simulink model "mqam_2020a"  (R2020a)
settings: Solver=VariableStepAuto  StartTime=0.0  StopTime=10  RelTol=1e-3
PreLoadFcn:
  | %%% model parameters %%%
  | 
  | Rb = 10e6; % bit rate
  | Tb = 1/Rb; % bit interval
  | 
  | M = 256; % constelation alphabet
  | Nb = log2(M); % number of bit per symbol
  | 
  | Rsy = Rb/Nb; % symbol rate
  | Tsy = 1/Rsy; % symbol time
  | 
  | N = 100; % number of samples per symbol
  | 
  | Rsamp = N*Rsy; % sampling rate
  | Tsamp = 1/Rsamp; % samping interval
  | 
  | fc = 1/(4*Tsamp); % carrier frequency
  | 
  | Eg = 5; % baseband pulse shaping energy
  | 
  | %%% gray code mapper %%%
  | 
  | gray_codes = get_gray_codes(Nb/2);
  | 
  | gray_cont = containers.Map % container
  | for i=1:size(gray_codes,2)
  |   binary_str = num2str(flip(gray_codes(:,i)'));
  |   binary_str(binary_str == ' ') = '';
  |   gray_cont(binary_str) = (i-1)*2 - (sqrt(M) - 1);
  | end
  | 
  | %%% define the basbase shaping filter gain %%%
  | aux = rcosdesign(0.2, 4, N, 'normal');
  | Kg = 1/sqrt(trapz(Tsamp, aux.^2)); % filter gain so that the filter energy be normalized to unity
InitFcn:
  | phi = 0; % phase offset
undefined symbols (not defined in the file or in its folder): DiscIntNeverNeededParam, magnitude
libraries: dspsrcs4 x2, commchan3 x1, commfilt2 x1, commrandsrc3 x1, dsparch4 x1, commsink2 x1
settings Model: Creator=tapyu  LastModifiedBy=tapyu
settings DebuggingCC: UnconnectedInputMsg=none  UnconnectedOutputMsg=none  UnconnectedLineMsg=none  SFMachineParentedDataDiag=error

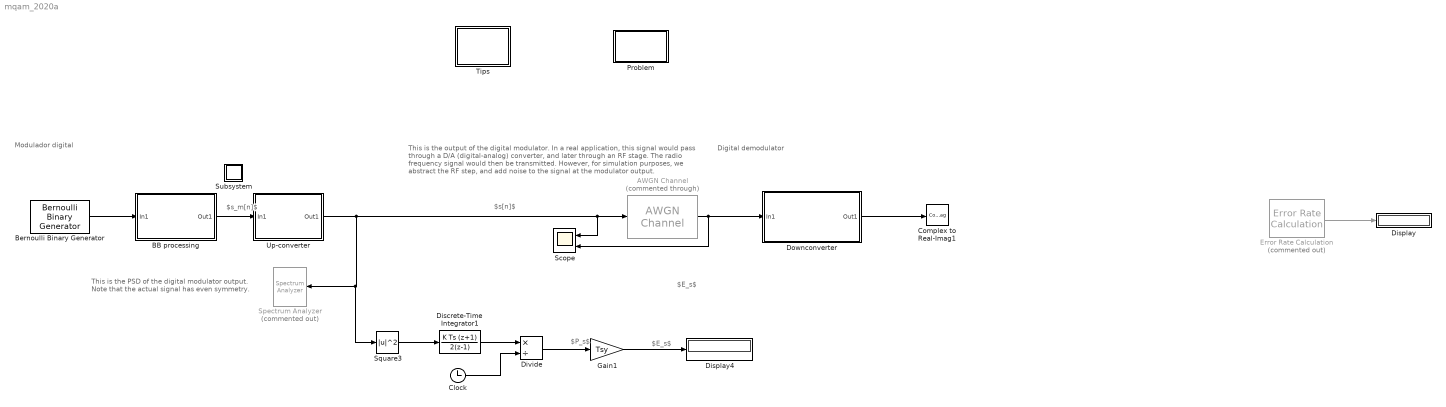
== system mqam_2020a ==
  note: Digital demodulator
  note: This is the output of the digital modulator. In a real application, this signal would
      | pass through a D/A (digital-analog) converter, and later through an RF stage.
      | The radio frequency signal would then be transmitted. However, for simulation
      | purposes, we abstract the RF step, and add noise to the signal at the modulator
      | output.
  note: $s[n]$
  note: This is the PSD of the digital modulator output.
      | Note that the actual signal has even symmetry.
  note: Modulador digital
  note: $s_m[n]$
  note: $E_s$
  note: $P_s$
  note: $E_s$
  AWGN Channel : commchan3/AWGN Channel  Commented=through  InputProcessing=Columns as channels (frame based)  seed=67  noiseMode="Signal to noise ratio  (Eb/No)"  EbNodB=10  EsNodB=10  SNRdB=10  bitsPerSym=sqrt(M)  Ps=1  Tsym=Tb  variance=1
  BB processing : Subsystem
  Bernoulli Binary Generator : commrandsrc3/Bernoulli Binary Generator  ProbabilityOfZero=0.5  SeedSource=Auto  Seed=0  SampleTime=Tb  SamplesPerFrame=1  OutputDataType=double  SimulateUsing=Interpreted execution
  Clock : Clock
  Complex to Real-Imag1 : ComplexToRealImag
  Discrete-Time Integrator1 : DiscreteIntegrator  IntegratorMethod=Integration: Trapezoidal  SampleTime=-1  ICPrevOutput=DiscIntNeverNeededParam  ICPrevScaledInput=DiscIntNeverNeededParam
  Display : Display
  Display4 : Display
  Divide : Product  Inputs=*/
  Downconverter : Subsystem
  Error Rate Calculation : commsink2/Error Rate Calculation  Commented=on  N=0  st_delay=0  cp_mode=Entire frame  subframe=[]  PMode=Port  WsName=ErrorVec  RsMode2=off  stop=off  numErr=100  maxBits=1e6
  Gain1 : Gain  Gain=Tsy
  Problem : Subsystem
  Scope : Scope  NumInputPorts=2
  Spectrum Analyzer : SpectrumAnalyzer  Commented=on
  Square3 : Math  Operator=magnitude^2  SaturateOnIntegerOverflow=on
  Subsystem : Subsystem
  Tips : Subsystem
  Up-converter : Subsystem
  wires:
  BB processing/1(Out1) -> Up-converter/1(In1)
  AWGN Channel/1 -> Downconverter/1(In1), Scope/2
  Error Rate Calculation/1 -> Display/1
  Downconverter/1(Out1) -> Complex to Real-Imag1/1
  Bernoulli Binary Generator/1 -> BB processing/1(In1)
  Gain1/1 -> Display4/1
  Clock/1 -> Divide/2
  Divide/1 -> Gain1/1
  Discrete-Time Integrator1/1 -> Divide/1
  Up-converter/1(Out1) -> Square3/1, Spectrum Analyzer/1, Scope/1, AWGN Channel/1
  Square3/1 -> Discrete-Time Integrator1/1

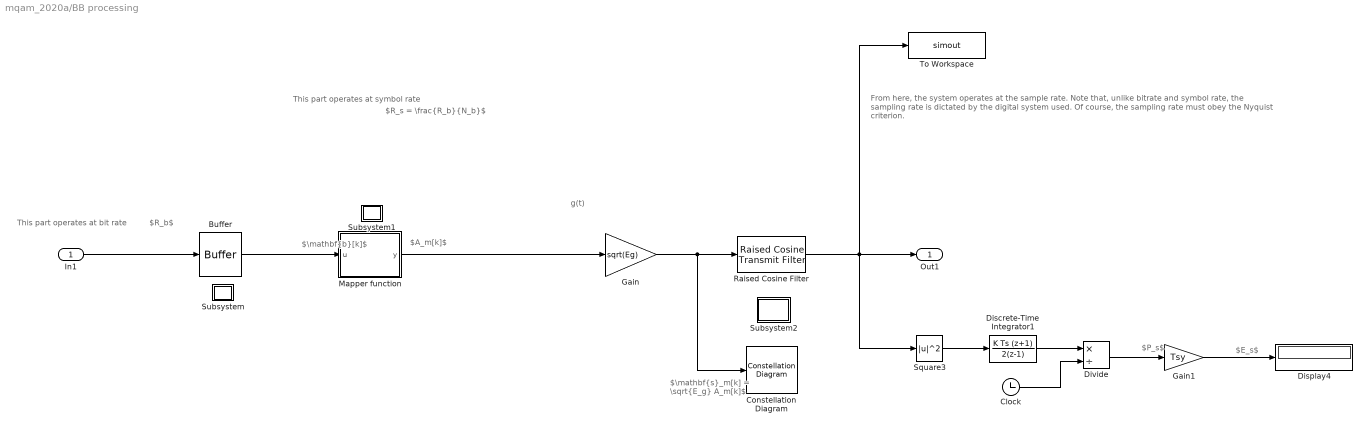
== system mqam_2020a/BB processing ==
  note: $P_s$
  note: g(t)
  note: From here, the system operates at the sample rate. Note that, unlike bitrate and symbol rate,
      | the sampling rate is dictated by the digital system used. Of course, the sampling rate must
      | obey the Nyquist criterion.
  note: $R_s = \frac{R_b}{N_b}$
  note: This part operates
      | at symbol rate
  note: $R_b$
  note: This part operates at bit rate
  note: $A_m[k]$
  note: $\mathbf{b}[k]$
  note: $\mathbf{s}_m[k] = \sqrt{E_g} A_m[k]$
  note: $E_s$
  In1 : Inport
  Buffer : Buffer  N=Nb  OutputFrames=off
  Clock : Clock
  Constellation Diagram : ConstellationDiagram
  Discrete-Time Integrator1 : DiscreteIntegrator  IntegratorMethod=Integration: Trapezoidal  SampleTime=-1  ICPrevOutput=DiscIntNeverNeededParam  ICPrevScaledInput=DiscIntNeverNeededParam
  Display4 : Display
  Divide : Product  Inputs=*/
  Gain : Gain  Gain=sqrt(Eg)
  Gain1 : Gain  Gain=Tsy
  Mapper function : MATLAB Function  TreatAsAtomicUnit=on
  Raised Cosine Filter : commfilt2/Raised Cosine Transmit Filter  filtType=Normal  R=0.2  filtSpan=4  N=N  filterGain=Kg  RateOptions=Allow multirate processing  framing=Mute  checkCoeff=on  variableName=rcTxFilt  checkGain=Normalized  sampMode=Mute  saveAsFlag=0  currentFiltSpan=4  D=(4)/2  launchFVT=on  roundingMode=Floor  overflowMode=off  coeffDataTypeStr=Inherit: Same word length as input  coeffMin=[]  coeffMax=[]  coeffLastDataTypeStr=Inherit: Same word length as input  outputDataTypeStr=Inherit: Same as accumulator  outputMin=[]  outputMax=[]  outputLastDataTypeStr=Inherit: Same as accumulator
  Square3 : Math  Operator=magnitude^2  SaturateOnIntegerOverflow=on
  Subsystem : Subsystem
  Subsystem1 : Subsystem
  Subsystem2 : Subsystem
  To Workspace : ToWorkspace  VariableName=simout  SaveFormat=Timeseries  SampleTime=-1
  Out1 : Outport
  wires:
  Buffer/1 -> Mapper function/1(u)
  Mapper function/1(y) -> Gain/1
  In1/1 -> Buffer/1
  Raised Cosine Filter/1 -> To Workspace/1, Square3/1, Out1/1
  Gain/1 -> Raised Cosine Filter/1, Constellation Diagram/1
  Square3/1 -> Discrete-Time Integrator1/1
  Discrete-Time Integrator1/1 -> Divide/1
  Clock/1 -> Divide/2
  Divide/1 -> Gain1/1
  Gain1/1 -> Display4/1

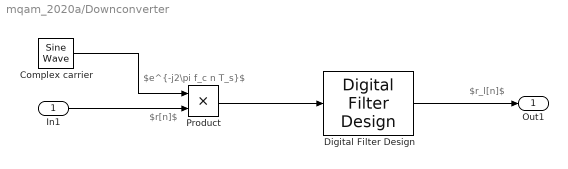
== system mqam_2020a/Downconverter ==
  note: $r[n]$
  note: $e^{-j2\pi f_c n T_s}$
  note: $r_l[n]$
  In1 : Inport
  Complex carrier : dspsrcs4/Sine Wave  Amplitude=sqrt(2)  Frequency=fc  Phase=0  SampleMode=Discrete  OutComplex=Complex  CompMethod=Trigonometric fcn  TableSize=Speed  SampleTime=Tsamp  SamplesPerFrame=1  ResetState=Restart at time zero  OutputFrames=off  dataType=double  wordLen=16  udDataType=sfix(16)  fracBitsMode=Best precision  numFracBits=15  OutDataTypeStr=double  LastOutDataTypeStr=double
  Digital Filter Design : dsparch4/Digital Filter Design  mwdsp_browser_bugfix_var=off
  Product : Product
  Out1 : Outport
  wires:
  In1/1 -> Product/2
  Complex carrier/1 -> Product/1
  Product/1 -> Digital Filter Design/1
  Digital Filter Design/1 -> Out1/1

== system mqam_2020a/Problem ==
  note: Bit rate:

== system mqam_2020a/Subsystem ==
  note: This is the complex envelope, also called the low-pass equivalent of the modulation scheme.

== system mqam_2020a/Tips ==
  note: Tips:
      |
      | - Go to debug->information overlays to set/unset visual indicators (called overlays). The main ones are: colors, timing legend, signals dimensions, base data types
      | - Go to modeling->model explorer->mqam->callbacks->PreLoadFnc to see the variables declared in this Simulink model. They are visible in the workspace area of the main window. In addition they can also be changed in the command window.

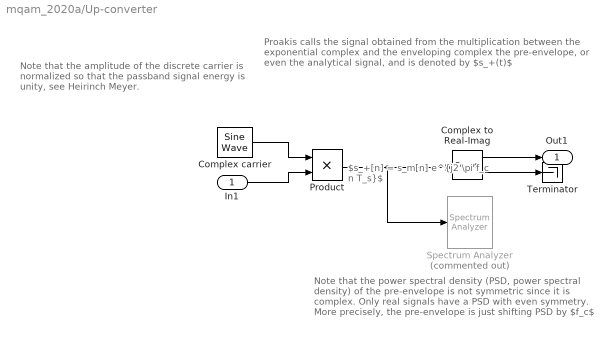
== system mqam_2020a/Up-converter ==
  note: Note that the amplitude of the discrete carrier is
      | normalized so that the passband signal energy
      | is unity, see Heirinch Meyer.
  note: Note that the power spectral density (PSD, power spectral density) of the pre-envelope is not symmetric since it is complex.
      |
      | Only real signals have a PSD with even symmetry. More precisely, the pre-envelope is just shifting PSD by $f_c$
  note: Proakis calls the signal obtained from the multiplication between the
      | exponential complex and the enveloping complex the pre-envelope,
      | or even the analytical signal, and is denoted by $s_+(t)$
  note: $s_+[n] = s_m[n] e^{j2 \pi f_c n T_s}$
  In1 : Inport
  Complex carrier : dspsrcs4/Sine Wave  Amplitude=sqrt(2)  Frequency=fc  Phase=0  SampleMode=Discrete  OutComplex=Complex  CompMethod=Trigonometric fcn  TableSize=Speed  SampleTime=Tsamp  SamplesPerFrame=1  ResetState=Restart at time zero  OutputFrames=off  dataType=double  wordLen=16  udDataType=sfix(16)  fracBitsMode=Best precision  numFracBits=15  OutDataTypeStr=double  LastOutDataTypeStr=double
  Complex to Real-Imag : ComplexToRealImag
  Product : Product
  Spectrum Analyzer : SpectrumAnalyzer  Commented=on
  Terminator : Terminator
  Out1 : Outport
  wires:
  Complex carrier/1 -> Product/1
  In1/1 -> Product/2
  Complex to Real-Imag/1 -> Out1/1
  Product/1 -> Spectrum Analyzer/1, Complex to Real-Imag/1
  Complex to Real-Imag/2 -> Terminator/1

== system mqam_2020a/BB processing/Subsystem ==
  note: The bitstream operates at a rate of $R_b = 10 Mbps$ . The first task is to transform the stream bit into a vector, $\mathbf{b}[k] \in \mathbb{R}^{K}$ , where $k \in \mathbb{N}_+$ is the $k$ th set of $K = \log_2 (M)$ bits

== system mqam_2020a/BB processing/Subsystem1 ==
  note: Each sequence of $K = \log_2(M)$ bit is mapped (using Gray code) to a complex symbol, $A_m[k]$ , where $m \in \{1,2,\cdots,M\}$ is the $m$ th complex symbol of the alphabet, and $k \in \mathbb{N}_+$ is the $k$ th transmitted symbol

== system mqam_2020a/BB processing/Subsystem2 ==
  note: The complex symbol is up-sampled, which changes the sample rate of the modulator from $k$ to $n$ through a method known as zero-padding. Between each complex symbol, $N-1$ zeros are added. Therefore, the number of samples by symbols is $N$ . After that, the symbol train passes through a FIR filter whose impulse response, $g[n]$ , is the discrete function of raised cosine, where $n\in \mathbb{N}_+$ indicates the discrete time instant of the signal that operates at the sampling rate, $R=N R_s$ . The filter output signal for the kth transmitted symbol is given by $s[n] = A_m[k] g[n]$ . This signal is commonly referred to as the complex envelope. Click on the raised cosine filter block->view filter response and note the following points:
      |
      | - The raised cosine filter's impulse response is actually a truncated version of it into 4 symbol intervals (recall that each symbol interval contains $N$ sampled). The reason for this is feasibility at the time of implementation: it is not possible to define a FIR filter with an impulse response of infinite duration, so it is necessary to truncate it. Note that the effect of time truncation leads to a distortion of the frequency response of the FIR filter. There is then a compromise term (trade-off) between the size of the truncation window and the level of distortion of the frequency response.
      |
      | - Note that, although there is overlap between the neighboring symbols, the null interference in the optimal decimation instants: count $N$ samples from the peak instant and see which pulse crosses the zero value at these instants. This is because the raised cosine pulse respects the Nyquist criterion of non-ISI.
      |
      | - The amplitude of the raised cosine is modified in such a way that its energy is normalized. The energy of the baseband signal (denotes as $E_g$ ) is inserted separately as a gain of $\sqrt{E_g}$

== matlab function mqam_2020a/BB processing/Mapper function ==
  data: u input; y output; gray_codes parameter; M parameter
function y = fcn(u, gray_codes, M)

v = [u(1:end/2), u(end/2+1:end)];
w = zeros(2,1);

for i = 1:2
    for j = 1:size(gray_codes,2)
        if all(gray_codes(:,j) == v(:,i))
            w(i) = (j-1)*2 - (sqrt(M) - 1);
            break
        end
    end
end

y = w(1) + 1j*w(2);
end
